simulink model "RCAM_Sim"  (R2019b)
settings: Solver=VariableStepAuto  StartTime=0.0  StopTime=TF  RelTol=1e-3
values from neighbouring files (symbols this model uses):
  x0 = [85 ... (first row only)    [RCAM_Init.m]
undefined symbols (not defined in the file or in its folder): RCAM_Model
settings Model: Creator=wilson  LastModifiedBy=wilson

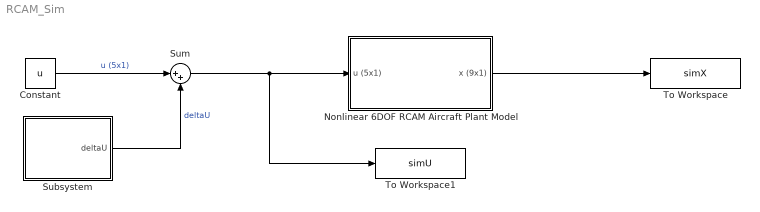
== system RCAM_Sim ==
  Constant : Constant  Value=u
  Nonlinear 6DOF RCAM Aircraft Plant Model : Subsystem
  Subsystem : Subsystem
  Sum : Sum  Inputs=|++
  To Workspace : ToWorkspace  VariableName=simX  SaveFormat=Timeseries  SampleTime=-1
      settings: Save2DSignal=2-D array (concatenate along first dimension)
  To Workspace1 : ToWorkspace  VariableName=simU  SaveFormat=Timeseries  SampleTime=-1
      settings: Save2DSignal=2-D array (concatenate along first dimension)
  wires:
  Nonlinear 6DOF RCAM Aircraft Plant Model/1(x (9x1)) -> To Workspace/1
  Constant/1 -> Sum/1  "u (5x1)"
  Sum/1 -> To Workspace1/1, Nonlinear 6DOF RCAM Aircraft Plant Model/1(u (5x1))
  Subsystem/1(deltaU) -> Sum/2  "deltaU"

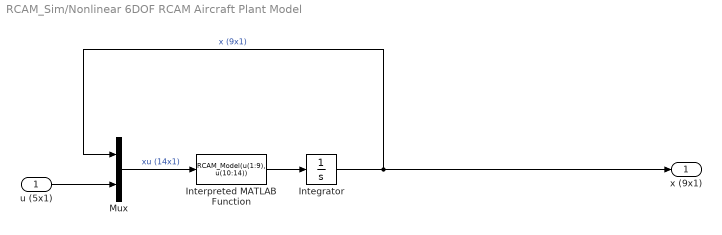
== system RCAM_Sim/Nonlinear 6DOF RCAM Aircraft Plant Model ==
  u (5x1) : Inport
  Integrator : Integrator  InitialCondition=x0
  Interpreted MATLAB Function : MATLABFcn  MATLABFcn=RCAM_Model(u(1:9), u(10:14))
  Mux : Mux  Inputs=2
  x (9x1) : Outport
  wires:
  Integrator/1 -> x (9x1)/1, Mux/1  "x (9x1)"
  Mux/1 -> Interpreted MATLAB Function/1  "xu (14x1)"
  u (5x1)/1 -> Mux/2
  Interpreted MATLAB Function/1 -> Integrator/1

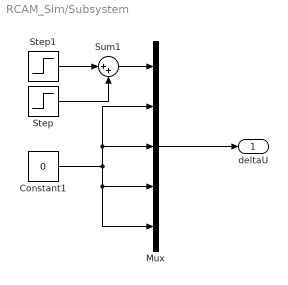
== system RCAM_Sim/Subsystem ==
  Constant1 : Constant  Value=0
  Mux : Mux  Inputs=5
  Step : Step  Time=32  After=-5*pi/180  SampleTime=0
  Step1 : Step  Time=30  After=5*pi/180  SampleTime=0
  Sum1 : Sum  Inputs=|++
  deltaU : Outport
  wires:
  Step/1 -> Sum1/2
  Constant1/1 -> Mux/2, Mux/3, Mux/5, Mux/4
  Step1/1 -> Sum1/1
  Sum1/1 -> Mux/1
  Mux/1 -> deltaU/1
